simulink model "discrete_buckconverter"  (R2022a)
settings: Solver=ode23t  StartTime=0.0  StopTime=t_sim  MaxStep=1e-6  RelTol=1e-12
values from neighbouring files (symbols this model uses):
  C = 200e-6    (= 0.0002)    [buck_parameters2.m]    (also in parameter_buck.m = 0.0001; synchronousBuck_converter_parameters.m = 0.0001)
  I_L_int = 1    [buck_con_DVMC_simulation.m]    (also in buck_parameters2.m = 0; parameter_buck.m = 0; synchronousBuck_converter_parameters.m = 0)
  K_dd = 20    [buck_con_DVMC_simulation.m]    (also in buck_converter_pid_control.m = K_da/T; parameter_buck.m = 10)
  K_id = 0.3    [buck_con_DVMC_simulation.m]    (also in buck_converter_pid_control.m = K_ia*T; parameter_buck.m = 0.05)
  K_pd = 10    [buck_con_DVMC_simulation.m]    (also in buck_converter_pid_control.m = K_pa; parameter_buck.m)
  L = 0.5e-6    (= 5e-07)    [buck_parameters2.m]    (also in parameter_buck.m = 2e-06; synchronousBuck_converter_parameters.m = 2e-06)
  R = 1    [Buck_converter_Discerete_TF_model.m]    (also in buck_con_DVMC_simulation.m; buck_converter_CT_TF_model.m; buck_converter_pid_control.m; parameter_buck.m = 0.5)
  r_C = 3e-3    (= 0.003)    [buck_parameters2.m]    (also in parameter_buck.m = 0.005; synchronousBuck_converter_parameters.m = 0.005)
  r_d = 10e-3    (= 0.01)    [buck_parameters2.m]    (also in parameter_buck.m)
  r_L = 5e-3    (= 0.005)    [buck_parameters2.m]    (also in parameter_buck.m = 0.01; synchronousBuck_converter_parameters.m = 0.01)
  T = 1e-6    (= 1e-06)    [buck_parameters2.m]    (also in parameter_buck.m; synchronousBuck_converter_parameters.m)
  V_C_int = 0.99    [buck_con_DVMC_simulation.m]    (also in buck_parameters2.m = 0; parameter_buck.m = 0; synchronousBuck_converter_parameters.m = 0)
  V_d = 0.55    [buck_parameters2.m]    (also in parameter_buck.m = 0.7)
  Vin = 12    [buck_parameters2.m]    (also in parameter_buck.m; synchronousBuck_converter_parameters.m)
  Vref = 1    [buck_parameters2.m]    (also in parameter_buck.m = 3.3)
libraries: slpidlib x1, simulink x1, simulink_extras x1
settings Model: Creator=Aravind  LastModifiedBy=Aravind

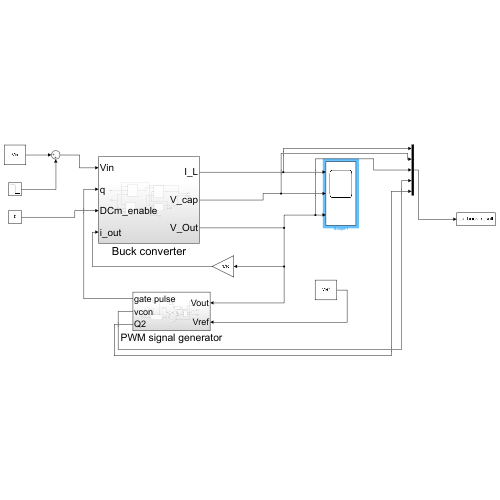
[thumbnail: Simulink's stored preview of the top-level diagram]
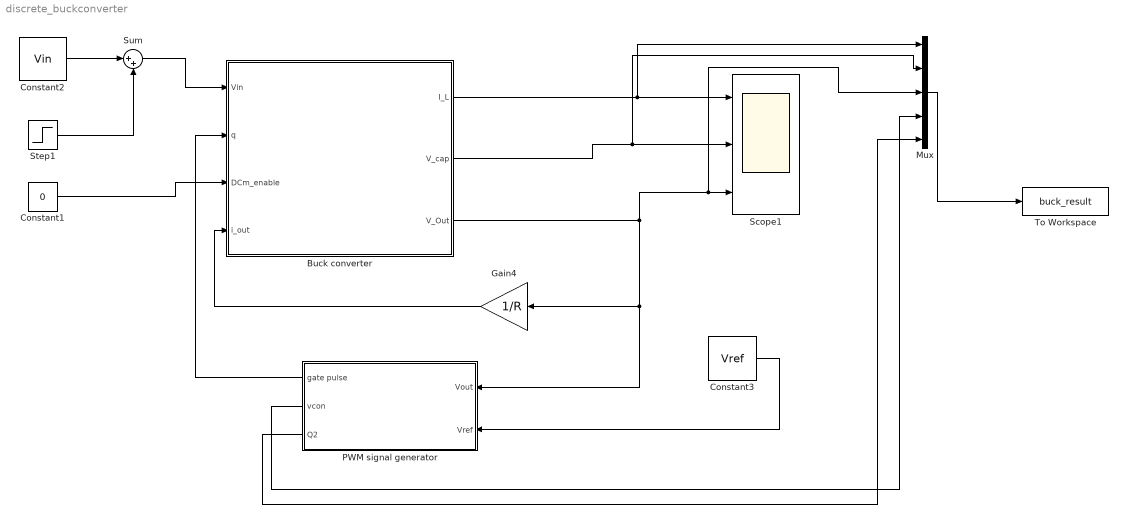
== system discrete_buckconverter ==
  Buck converter : Subsystem
  Constant1 : Constant  Value=0
  Constant2 : Constant  Value=Vin
  Constant3 : Constant  Value=Vref
  Gain4 : Gain  Gain=1/R
  Mux : Mux  Inputs=5
  PWM signal generator : Subsystem
  Scope1 : Scope  NumInputPorts=3
  Step1 : Step  Time=5  After=-4  SampleTime=0
  Sum : Sum  Inputs=|++
  To Workspace : ToWorkspace  VariableName=buck_result  SaveFormat=Structure With Time  SampleTime=-1
  wires:
  PWM signal generator/1(gate pulse) -> Buck converter/2(q)
  Buck converter/3(V_Out) -> Gain4/1, PWM signal generator/1(Vout), Mux/3, Scope1/3
  Constant2/1 -> Sum/1
  Constant1/1 -> Buck converter/3(DCm_enable)
  Sum/1 -> Buck converter/1(Vin)
  Step1/1 -> Sum/2
  Constant3/1 -> PWM signal generator/2(Vref)
  Buck converter/1(I_L) -> Mux/1, Scope1/1
  Gain4/1 -> Buck converter/4(i_out)
  PWM signal generator/2(vcon) -> Mux/4
  PWM signal generator/3(Q2) -> Mux/5
  Mux/1 -> To Workspace/1
  Buck converter/2(V_cap) -> Mux/2, Scope1/2

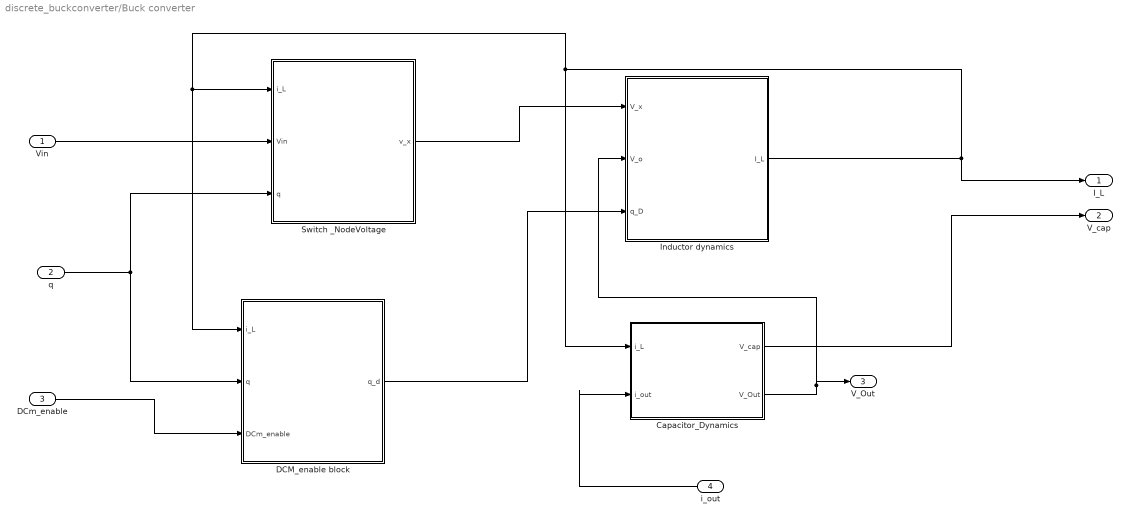
== system discrete_buckconverter/Buck converter ==
  Vin : Inport
  q : Inport  Port=2
  DCm_enable : Inport  Port=3
  i_out : Inport  Port=4
  Capacitor_Dynamics : Subsystem
  DCM_enable block : Subsystem
  Inductor dynamics : Subsystem
  Switch _NodeVoltage : Subsystem
  I_L : Outport
  V_cap : Outport  Port=2
  V_Out : Outport  Port=3
  wires:
  Vin/1 -> Switch _NodeVoltage/2(Vin)
  Capacitor_Dynamics/2(V_Out) -> Inductor dynamics/2(V_o), V_Out/1
  q/1 -> Switch _NodeVoltage/3(q), DCM_enable block/2(q)
  Inductor dynamics/1(I_L) -> I_L/1, Switch _NodeVoltage/1(i_L), DCM_enable block/1(i_L), Capacitor_Dynamics/1(i_L)
  DCm_enable/1 -> DCM_enable block/3(DCm_enable)
  Switch _NodeVoltage/1(v_x) -> Inductor dynamics/1(V_x)
  i_out/1 -> Capacitor_Dynamics/2(i_out)
  DCM_enable block/1(q_d) -> Inductor dynamics/3(q_D)
  Capacitor_Dynamics/1(V_cap) -> V_cap/1

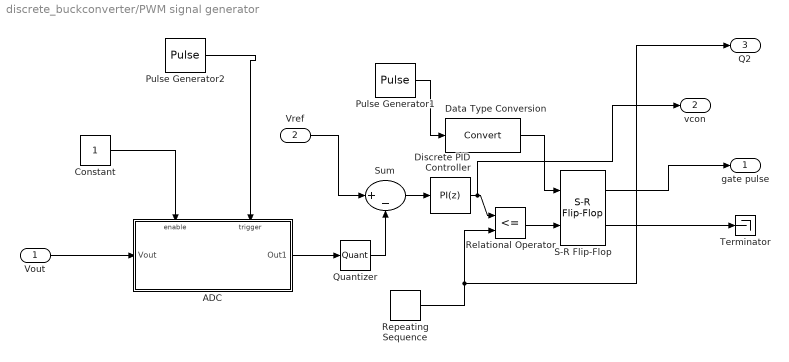
== system discrete_buckconverter/PWM signal generator ==
  Vout : Inport
  Vref : Inport  Port=2
  ADC : Subsystem  TreatAsAtomicUnit=on
  Constant : Constant
  Data Type Conversion : DataTypeConversion  OutMin=[0]  OutMax=[1]  SaturateOnIntegerOverflow=off  RndMeth=Floor
  Discrete PID Controller : slpidlib/PID Controller  Controller=PI  Form=Parallel  TimeDomain=Discrete-time  UseExternalTs=off  SampleTime=-1  IntegratorMethod=Forward Euler  FilterMethod=Forward Euler  ControllerParametersSource=internal  P=K_pd  I=K_id  UseKiTs=off  D=K_dd  N=100  UseFilter=on  TunerSelectOption=Transfer Function Based (PID Tuner App)  InitialConditionSource=internal  InitialConditionForIntegrator=0  InitialConditionForFilter=0  DifferentiatorICPrevScaledInput=0  ExternalReset=none  TrackingMode=off  Kt=1  LimitOutput=off  SatLimitsSource=internal  UpperSaturationLimit=inf  LowerSaturationLimit=-inf  LinearizeAsGain=off  AntiWindupMode=none  Kb=1  POutMin=[]  POutMax=[]  IOutMin=[]  IOutMax=[]  DOutMin=[]  DOutMax=[]  NOutMin=[]  NOutMax=[]  SumOutMin=[]  SumOutMax=[]  SaturationOutMin=[]  SaturationOutMax=[]  PParamMin=[]  PParamMax=[]  IParamMin=[]  IParamMax=[]  DParamMin=[]  DParamMax=[]  NParamMin=[]  NParamMax=[]  KbParamMin=[]  KbParamMax=[]  KtParamMin=[]  KtParamMax=[]  KbOutMin=[]  KbOutMax=[]  KtOutMin=[]  KtOutMax=[]  IntegratorOutMin=[]  IntegratorOutMax=[]  FilterOutMin=[]  FilterOutMax=[]  SumI1OutMin=[]  SumI1OutMax=[]  SumI2OutMin=[]  SumI2OutMax=[]  SumI3OutMin=[]  SumI3OutMax=[]  SumI4OutMin=[]  SumI4OutMax=[]  SumDOutMin=[]  SumDOutMax=[]  DifferentiatorOutMin=[]  DifferentiatorOutMax=[]  FilterDiffOutCoefMin=[]  FilterDiffOutCoefMax=[]  ReciprocalOutMin=[]  ReciprocalOutMax=[]  SumDenOutMin=[]  SumDenOutMax=[]  SumNumOutMin=[]  SumNumOutMax=[]  DivideOutMin=[]  DivideOutMax=[]  UdiffTsProdOutMin=[]  UdiffTsProdOutMax=[]  NTsProdOutMin=[]  NTsProdOutMax=[]  UintegralTsProdOutMin=[]  UintegralTsProdOutMax=[]  UngainTsProdOutMin=[]  UngainTsProdOutMax=[]  IntegratorContinuousStateAttributes=''  IntegratorStateMustResolveToSignalObject=off  IntegratorRTWStateStorageClass=Auto  FilterContinuousStateAttributes=''  FilterStateMustResolveToSignalObject=off  FilterRTWStateStorageClass=Auto  ParallelPVariant=InternalParameters  IdealPVariant=Disabled  IVariant=InternalParameters  DVariant=Disabled  IntegratorVariant=Discrete  SatVariant=Disabled  AWVariant=Passthrough  PCopyVariant=Disabled  TRVariant=Disabled  FdbkBlocksVariant=Forward  IdealPFdbkVariant=Disabled  SatFdbkVariant=Disabled  DerivativeFilterVariant=Disabled  NVariant=Disabled  NCopyVariant=Disabled_SignalSpec  FilterICVariant=Disabled  IntegratorICVariant=InternalICs  ExternalResetVariant=Disabled  TRSumVariant=Passthrough  SumFdbkVariant=Disabled  SumVariant=Sum_PI  TsampFilterVariant=InternalTs  TsampNgainVariant=Passthrough  TsampIntegralVariant=Passthrough  ExternalSaturationOutDataTypeStr=Inherit: Same as second input  aMode=0
  Pulse Generator1 : DiscretePulseGenerator  PulseType=Time based  Period=T  PulseWidth=50
  Pulse Generator2 : DiscretePulseGenerator  PulseType=Time based  Period=T  PulseWidth=50
  Quantizer : Quantizer  QuantizationInterval=0.001
  Relational Operator : RelationalOperator  Operator=<=  OutDataTypeStr=boolean  RndMeth=Simplest  InputSameDT=off
  Repeating Sequence : simulink/Sources/Repeating Sequence  rep_seq_t=[0 T]  rep_seq_y=[0 1]
  S-R Flip-Flop : simulink_extras/Flip Flops/S-R Flip-Flop  initial_condition=0
  Sum : Sum  Inputs=|+-
  Terminator : Terminator
  gate pulse : Outport
  vcon : Outport  Port=2
  Q2 : Outport  Port=3
  wires:
  S-R Flip-Flop/2 -> Terminator/1
  S-R Flip-Flop/1 -> gate pulse/1
  Data Type Conversion/1 -> S-R Flip-Flop/1
  Pulse Generator1/1 -> Data Type Conversion/1
  Pulse Generator2/1 -> ADC/Trigger
  Constant/1 -> ADC/Enable
  Vout/1 -> ADC/1(Vout)
  Vref/1 -> Sum/1
  Relational Operator/1 -> S-R Flip-Flop/2
  Sum/1 -> Discrete PID Controller/1
  Discrete PID Controller/1 -> vcon/1, Relational Operator/1
  ADC/1(Out1) -> Quantizer/1
  Quantizer/1 -> Sum/2
  Repeating Sequence/1 -> Q2/1, Relational Operator/2

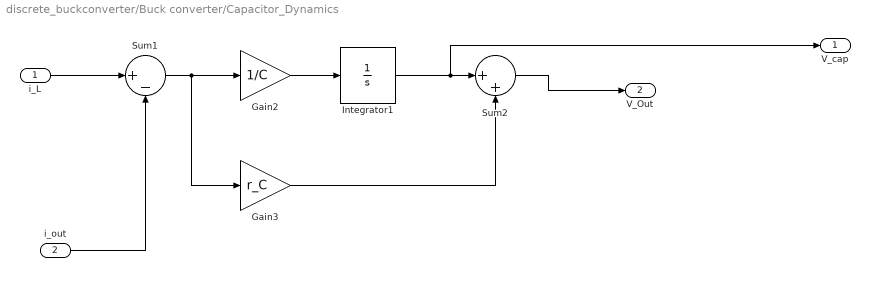
== system discrete_buckconverter/Buck converter/Capacitor_Dynamics ==
  i_L : Inport
  i_out : Inport  Port=2
  Gain2 : Gain  Gain=1/C
  Gain3 : Gain  Gain=r_C
  Integrator1 : Integrator  InitialCondition=V_C_int
  Sum1 : Sum  Inputs=|+-
  Sum2 : Sum  Inputs=|++
  V_cap : Outport
  V_Out : Outport  Port=2
  wires:
  Sum1/1 -> Gain2/1, Gain3/1
  Integrator1/1 -> V_cap/1, Sum2/1
  i_L/1 -> Sum1/1
  Sum2/1 -> V_Out/1
  i_out/1 -> Sum1/2
  Gain2/1 -> Integrator1/1
  Gain3/1 -> Sum2/2

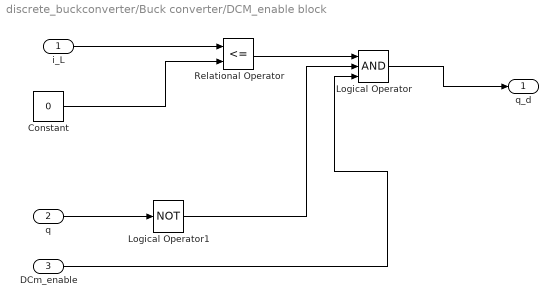
== system discrete_buckconverter/Buck converter/DCM_enable block ==
  i_L : Inport
  q : Inport  Port=2
  DCm_enable : Inport  Port=3
  Constant : Constant  Value=0
  Logical Operator : Logic  Inputs=3  AllPortsSameDT=off  OutDataTypeStr=boolean
  Logical Operator1 : Logic  Operator=NOT  Inputs=3  AllPortsSameDT=off  OutDataTypeStr=boolean
  Relational Operator : RelationalOperator  Operator=<=  OutDataTypeStr=boolean  RndMeth=Simplest  InputSameDT=off
  q_d : Outport
  wires:
  i_L/1 -> Relational Operator/1
  Constant/1 -> Relational Operator/2
  Relational Operator/1 -> Logical Operator/1
  Logical Operator1/1 -> Logical Operator/2
  q/1 -> Logical Operator1/1
  DCm_enable/1 -> Logical Operator/3
  Logical Operator/1 -> q_d/1

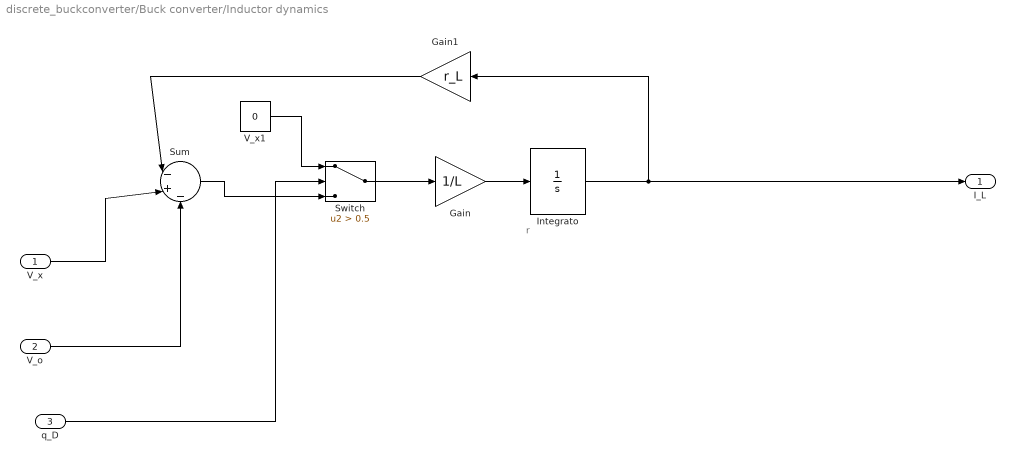
== system discrete_buckconverter/Buck converter/Inductor dynamics ==
  note: r
  V_x : Inport
  V_o : Inport  Port=2
  q_D : Inport  Port=3
  Gain : Gain  Gain=1/L
  Gain1 : Gain  Gain=r_L
  Integrato : Integrator  InitialCondition=I_L_int
  Sum : Sum  Inputs=|-+-
  Switch : Switch  Criteria=u2 > Threshold  Threshold=0.5  SaturateOnIntegerOverflow=off  InputSameDT=off
  V_x1 : Constant  Value=0
  I_L : Outport
  wires:
  q_D/1 -> Switch/2
  Gain1/1 -> Sum/1
  Integrato/1 -> I_L/1, Gain1/1
  Sum/1 -> Switch/3
  V_x1/1 -> Switch/1
  Gain/1 -> Integrato/1
  Switch/1 -> Gain/1
  V_x/1 -> Sum/2
  V_o/1 -> Sum/3

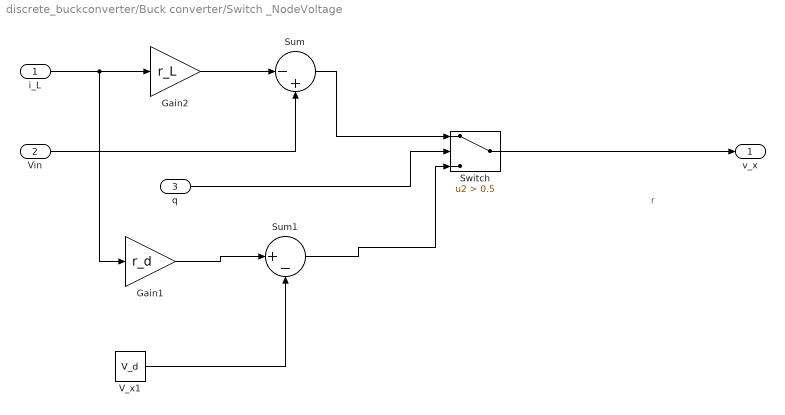
== system discrete_buckconverter/Buck converter/Switch _NodeVoltage ==
  note: r
  i_L : Inport
  Vin : Inport  Port=2
  q : Inport  Port=3
  Gain1 : Gain  Gain=r_d
  Gain2 : Gain  Gain=r_L
  Sum : Sum  Inputs=|-+
  Sum1 : Sum  Inputs=|+-
  Switch : Switch  Criteria=u2 > Threshold  Threshold=0.5  SaturateOnIntegerOverflow=off  InputSameDT=off
  V_x1 : Constant  Value=V_d
  v_x : Outport
  wires:
  Vin/1 -> Sum/2
  Switch/1 -> v_x/1
  q/1 -> Switch/2
  Gain2/1 -> Sum/1
  Sum/1 -> Switch/1
  V_x1/1 -> Sum1/2
  i_L/1 -> Gain1/1, Gain2/1
  Gain1/1 -> Sum1/1
  Sum1/1 -> Switch/3

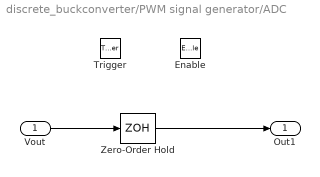
== system discrete_buckconverter/PWM signal generator/ADC ==
  Vout : Inport
  Enable : EnablePort
  Trigger : TriggerPort  VariantControl=(inherit)
  Zero-Order Hold : ZeroOrderHold  SampleTime=-1
  Out1 : Outport
  wires:
  Vout/1 -> Zero-Order Hold/1
  Zero-Order Hold/1 -> Out1/1
